simulink model "P4varianteinvariante"  (Simulink 7.1)
settings: Solver=ode45  StartTime=0.0  StopTime=10.0  RelTol=1e-3
settings Model: Creator=ALUNO  LastModifiedBy=ALUNO

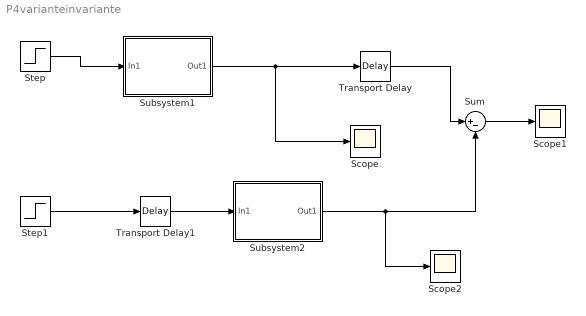
== system P4varianteinvariante ==
  Scope : Scope
  Scope1 : Scope
  Scope2 : Scope
      settings: SaveName=ScopeData2
  Step : Step  SampleTime=0
  Step1 : Step  SampleTime=0
  Subsystem1 : Subsystem
      mask Display: disp('Planta P4')
  Subsystem2 : Subsystem
      mask Display: disp('Planta P4')
  Sum : Sum  Inputs=|+-  OutDataType=sfix(16)  OutScaling=2^0
  Transport Delay : TransportDelay  DelayTime=2
  Transport Delay1 : TransportDelay  DelayTime=2
  wires:
  Step1/1 -> Transport Delay1/1
  Transport Delay1/1 -> Subsystem2/1(In1)
  Step/1 -> Subsystem1/1(In1)
  Subsystem1/1(Out1) -> Transport Delay/1, Scope/1
  Transport Delay/1 -> Sum/1
  Subsystem2/1(Out1) -> Sum/2, Scope2/1
  Sum/1 -> Scope1/1

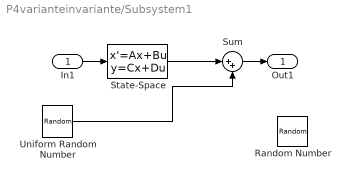
== system P4varianteinvariante/Subsystem1 ==
  In1 : Inport  OutDataType=sfix(16)  OutScaling=2^0
  Random Number : RandomNumber  Variance=0.25  SampleTime=0
  State-Space : StateSpace  A=[-1 -2;1 0]  B=[1; 0]  C="[0  2]"  D=0
  Sum : Sum  Inputs=|++  OutDataType=sfix(16)  OutScaling=2^0
  Uniform Random Number : UniformRandomNumber  Minimum=-0.25  Maximum=0.25  SampleTime=0
  Out1 : Outport  OutDataType=sfix(16)  OutScaling=2^0
  wires:
  State-Space/1 -> Sum/1
  In1/1 -> State-Space/1
  Sum/1 -> Out1/1
  Uniform Random Number/1 -> Sum/2

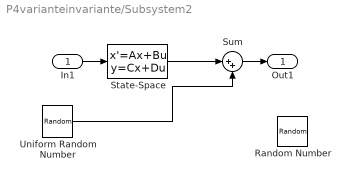
== system P4varianteinvariante/Subsystem2 ==
  In1 : Inport  OutDataType=sfix(16)  OutScaling=2^0
  Random Number : RandomNumber  Variance=0.25  SampleTime=0
  State-Space : StateSpace  A=[-1 -2;1 0]  B=[1; 0]  C="[0  2]"  D=0
  Sum : Sum  Inputs=|++  OutDataType=sfix(16)  OutScaling=2^0
  Uniform Random Number : UniformRandomNumber  Minimum=-0.25  Maximum=0.25  SampleTime=0
  Out1 : Outport  OutDataType=sfix(16)  OutScaling=2^0
  wires:
  State-Space/1 -> Sum/1
  In1/1 -> State-Space/1
  Sum/1 -> Out1/1
  Uniform Random Number/1 -> Sum/2
